simulink model "FOC"  (R2022a)
settings: Solver=VariableStepAuto  StartTime=0.0  StopTime=10.0  RelTol=1e-3
undefined symbols (not defined in the file): I_max, Ki_current, Kp_current, L_M_hat, magnitude, n_p, omega_1_N, psi_ref, R_R, R_R_hat, R_s, V_base, X_M_opt, X_sig_opt
libraries: eeTransforms x2, simulink x1, slpidlib x1
settings Model: Creator=Jakob  LastModifiedBy=Jakob

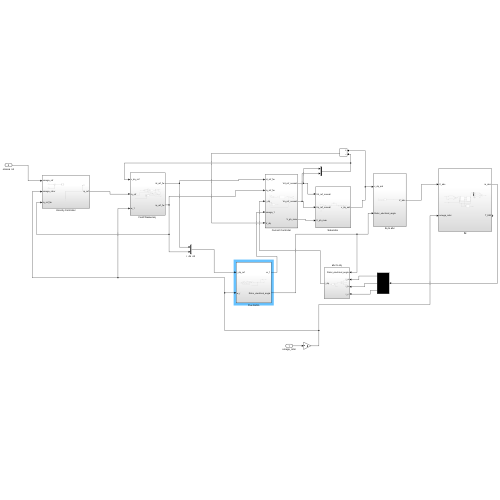
[thumbnail: Simulink's stored preview of the top-level diagram]
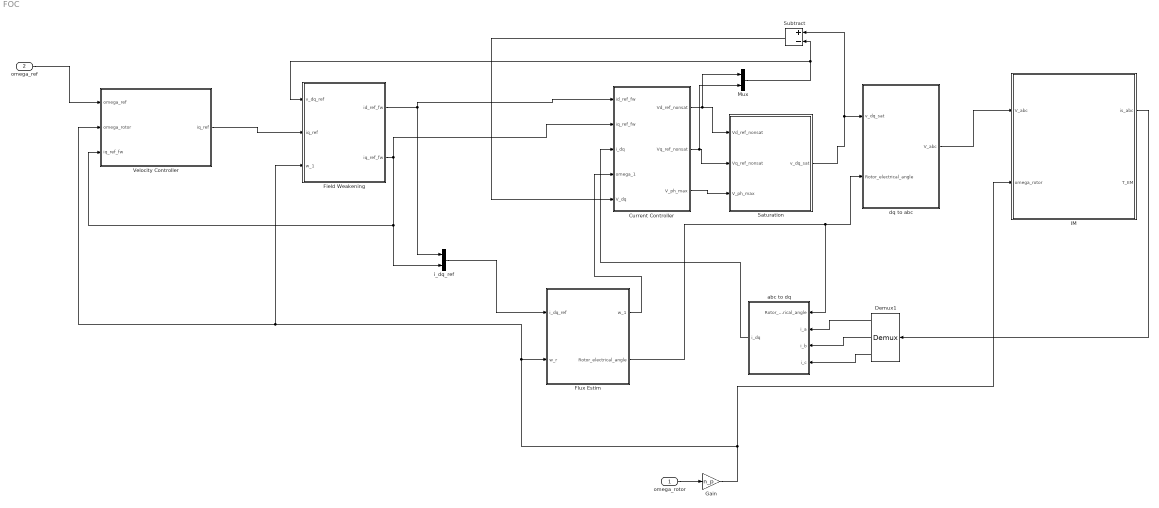
== system FOC ==
  omega_rotor : Inport
  omega_ref : Inport  Port=2
  Current Controller : Subsystem
  Demux1 : Demux  Outputs=3
  Field Weakening : Subsystem
  Flux Estim : Subsystem
  Gain : Gain  Gain=n_p
  IM : Subsystem
  Mux : Mux  Inputs=2
  Saturation : Subsystem
  Subtract : Sum  Inputs=+-
  Velocity Controller : Subsystem
  abc to dq : Subsystem
  dq to abc : Subsystem
  i_dq_ref : Mux  Inputs=2
  wires:
  dq to abc/1(V_abc) -> IM/1(V_abc)
  abc to dq/1(i_dq) -> Current Controller/3(i_dq)
  Current Controller/1(Vd_ref_nonsat) -> Mux/1, Saturation/1(Vd_ref_nonsat)
  Current Controller/2(Vq_ref_nonsat) -> Mux/2, Saturation/2(Vq_ref_nonsat)
  Current Controller/3(V_ph_max) -> Saturation/3(V_ph_max)
  Saturation/1(v_dq_sat) -> Subtract/1, dq to abc/1(v_dq_sat)
  Mux/1 -> Field Weakening/1(v_dq_ref), Subtract/2
  Subtract/1 -> Current Controller/5(V_dq)
  IM/1(is_abc) -> Demux1/1
  Demux1/1 -> abc to dq/2(i_a)
  Demux1/2 -> abc to dq/3(i_b)
  Demux1/3 -> abc to dq/4(i_c)
  omega_rotor/1 -> Gain/1
  omega_ref/1 -> Velocity Controller/1(omega_ref)
  Flux Estim/2(Rotor_electrical_angle) -> abc to dq/1(Rotor_electrical_angle), dq to abc/2(Rotor_electrical_angle)
  Flux Estim/1(w_1) -> Current Controller/4(omega_1)
  Gain/1 -> Flux Estim/2(w_r), Field Weakening/3(w_1), Velocity Controller/2(omega_rotor), IM/2(omega_rotor)
  Field Weakening/2(iq_ref_fw) -> Current Controller/2(iq_ref_fw), Velocity Controller/3(iq_ref_fw), i_dq_ref/2
  Velocity Controller/1(iq_ref) -> Field Weakening/2(iq_ref)
  Field Weakening/1(id_ref_fw) -> Current Controller/1(id_ref_fw), i_dq_ref/1
  i_dq_ref/1 -> Flux Estim/1(i_dq_ref)

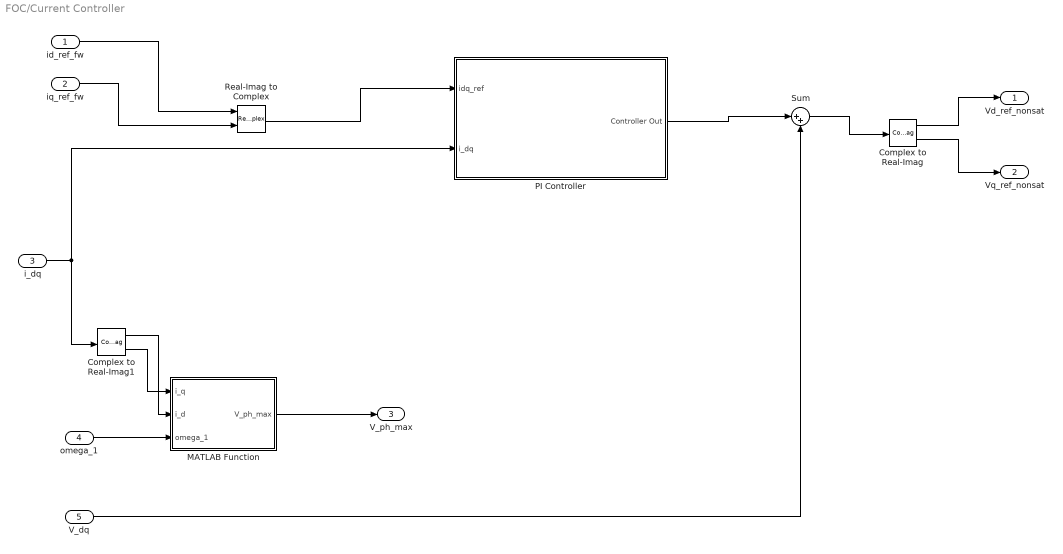
== system FOC/Current Controller ==
  id_ref_fw : Inport
  iq_ref_fw : Inport  Port=2
  i_dq : Inport  Port=3
  omega_1 : Inport  Port=4
  V_dq : Inport  Port=5
  Complex to Real-Imag : ComplexToRealImag
  Complex to Real-Imag1 : ComplexToRealImag
  MATLAB Function : MATLAB Function  TreatAsAtomicUnit=on
  PI Controller : Subsystem
  Real-Imag to Complex : RealImagToComplex
  Sum : Sum  Inputs=|++
  Vd_ref_nonsat : Outport
  Vq_ref_nonsat : Outport  Port=2
  V_ph_max : Outport  Port=3
  wires:
  i_dq/1 -> Complex to Real-Imag1/1, PI Controller/2(i_dq)
  Complex to Real-Imag1/1 -> MATLAB Function/2(i_d)
  Complex to Real-Imag1/2 -> MATLAB Function/1(i_q)
  omega_1/1 -> MATLAB Function/3(omega_1)
  id_ref_fw/1 -> Real-Imag to Complex/1
  iq_ref_fw/1 -> Real-Imag to Complex/2
  Real-Imag to Complex/1 -> PI Controller/1(idq_ref)
  PI Controller/1(Controller Out) -> Sum/1
  V_dq/1 -> Sum/2
  Sum/1 -> Complex to Real-Imag/1
  Complex to Real-Imag/1 -> Vd_ref_nonsat/1
  Complex to Real-Imag/2 -> Vq_ref_nonsat/1
  MATLAB Function/1(V_ph_max) -> V_ph_max/1

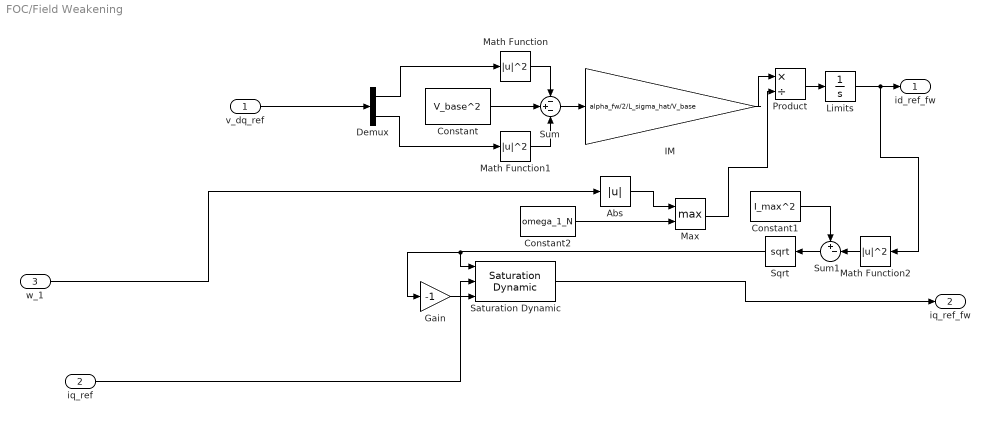
== system FOC/Field Weakening ==
  v_dq_ref : Inport
  iq_ref : Inport  Port=2
  w_1 : Inport  Port=3
  Abs : Abs  SaturateOnIntegerOverflow=off
  Constant : Constant  Value=V_base^2
  Constant1 : Constant  Value=I_max^2
  Constant2 : Constant  Value=omega_1_N
  Demux : Demux  Outputs=2
  Gain : Gain  Gain=-1
  IM : Gain  Gain=alpha_fw/2/L_sigma_hat/V_base
  Limits : Integrator  LimitOutput=on  UpperSaturationLimit=psi_ref/L_M_hat  LowerSaturationLimit=0.1*psi_ref/L_M_hat
  Math Function : Math  Operator=magnitude^2
  Math Function1 : Math  Operator=magnitude^2
  Math Function2 : Math  Operator=magnitude^2
  Max : MinMax  Function=max  Inputs=2
  Product : Product  Inputs=*/
  Saturation Dynamic : simulink/Discontinuities/Saturation Dynamic  OutMin=[]  OutMax=[]  OutDataTypeStr=Inherit: Same as second input  OutDataType=fixdt(1, 16)  OutScaling=2^-10  DoSatur=off
  Sqrt : Sqrt
  Sum : Sum  Inputs=-+-
  Sum1 : Sum  Inputs=+-|
  id_ref_fw : Outport
  iq_ref_fw : Outport  Port=2
  wires:
  Abs/1 -> Max/1
  Sum1/1 -> Sqrt/1
  Max/1 -> Product/2
  Math Function2/1 -> Sum1/2
  w_1/1 -> Abs/1
  v_dq_ref/1 -> Demux/1
  Math Function1/1 -> Sum/3
  Product/1 -> Limits/1
  Sqrt/1 -> Gain/1, Saturation Dynamic/1
  Gain/1 -> Saturation Dynamic/3
  Constant1/1 -> Sum1/1
  Constant2/1 -> Max/2
  Saturation Dynamic/1 -> iq_ref_fw/1
  Demux/2 -> Math Function1/1
  Limits/1 -> id_ref_fw/1, Math Function2/1
  Math Function/1 -> Sum/1
  IM/1 -> Product/1
  Sum/1 -> IM/1
  iq_ref/1 -> Saturation Dynamic/2
  Constant/1 -> Sum/2
  Demux/1 -> Math Function/1

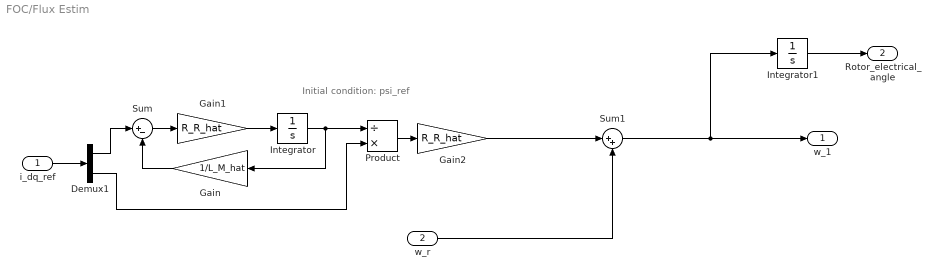
== system FOC/Flux Estim ==
  note: Initial condition: psi_ref
  i_dq_ref : Inport
  w_r : Inport  Port=2
  Demux1 : Demux  Outputs=2
  Gain : Gain  Gain=1/L_M_hat
  Gain1 : Gain  Gain=R_R_hat
  Gain2 : Gain  Gain=R_R_hat
  Integrator : Integrator  InitialCondition=psi_ref
  Integrator1 : Integrator
  Product : Product  Inputs=/*
  Sum : Sum  Inputs=|+-
  Sum1 : Sum  Inputs=|++
  w_1 : Outport
  Rotor_electrical_angle : Outport  Port=2
  wires:
  Gain1/1 -> Integrator/1
  Sum1/1 -> Integrator1/1, w_1/1
  Product/1 -> Gain2/1
  i_dq_ref/1 -> Demux1/1
  Demux1/1 -> Sum/1
  Demux1/2 -> Product/2
  Integrator/1 -> Gain/1, Product/1
  Gain/1 -> Sum/2
  Sum/1 -> Gain1/1
  Gain2/1 -> Sum1/1
  w_r/1 -> Sum1/2
  Integrator1/1 -> Rotor_electrical_angle/1

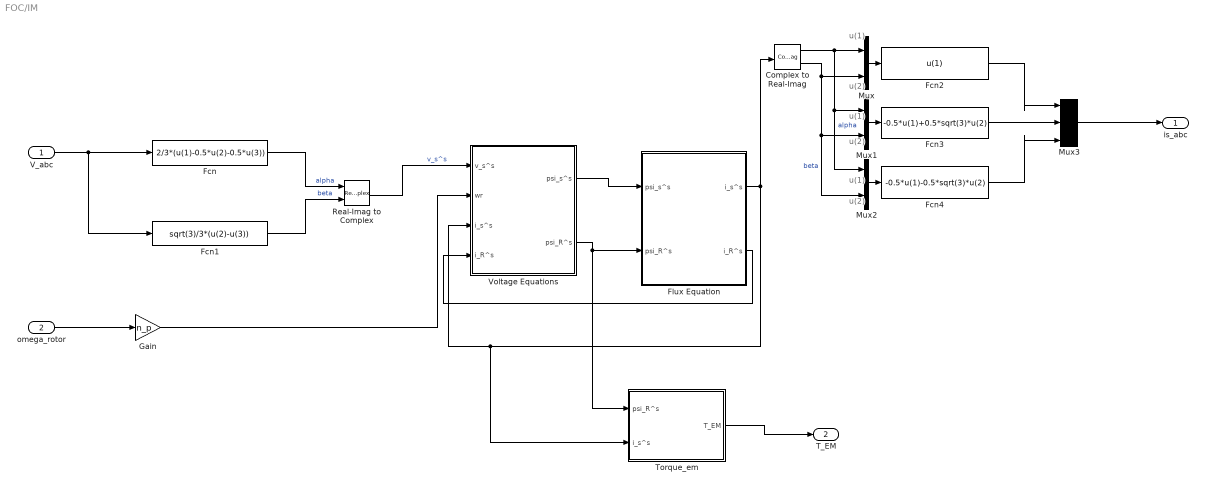
== system FOC/IM ==
  note: u(1)
  note: u(2)
  note: u(2)
  note: u(2)
  note: u(1)
  note: u(1)
  V_abc : Inport
  omega_rotor : Inport  Port=2
  Complex to Real-Imag : ComplexToRealImag
  Fcn : Fcn  Expr=2/3*(u(1)-0.5*u(2)-0.5*u(3))
  Fcn1 : Fcn  Expr=sqrt(3)/3*(u(2)-u(3))
  Fcn2 : Fcn  Expr=u(1)
  Fcn3 : Fcn  Expr=-0.5*u(1)+0.5*sqrt(3)*u(2)
  Fcn4 : Fcn  Expr=-0.5*u(1)-0.5*sqrt(3)*u(2)
  Flux Equation : Subsystem
  Gain : Gain  Gain=n_p
  Mux : Mux  Inputs=2
  Mux1 : Mux  Inputs=2
  Mux2 : Mux  Inputs=2
  Mux3 : Mux  Inputs=3
  Real-Imag to Complex : RealImagToComplex
  Torque_em : Subsystem
  Voltage Equations : Subsystem
  is_abc : Outport
  T_EM : Outport  Port=2
  wires:
  V_abc/1 -> Fcn1/1, Fcn/1
  Fcn/1 -> Real-Imag to Complex/1  "alpha"
  Fcn1/1 -> Real-Imag to Complex/2  "beta"
  Real-Imag to Complex/1 -> Voltage Equations/1(v_s^s)  "v_s^s"
  omega_rotor/1 -> Gain/1
  Gain/1 -> Voltage Equations/2(wr)
  Voltage Equations/1(psi_s^s) -> Flux Equation/1(psi_s^s)
  Voltage Equations/2(psi_R^s) -> Torque_em/1(psi_R^s), Flux Equation/2(psi_R^s)
  Complex to Real-Imag/1 -> Mux2/1, Mux1/1, Mux/1  "alpha"
  Mux/1 -> Fcn2/1
  Complex to Real-Imag/2 -> Mux2/2, Mux1/2, Mux/2  "beta"
  Mux2/1 -> Fcn4/1
  Flux Equation/1(i_s^s) -> Complex to Real-Imag/1, Torque_em/2(i_s^s), Voltage Equations/3(i_s^s)
  Mux1/1 -> Fcn3/1
  Fcn4/1 -> Mux3/3
  Fcn3/1 -> Mux3/2
  Fcn2/1 -> Mux3/1
  Mux3/1 -> is_abc/1
  Flux Equation/2(i_R^s) -> Voltage Equations/4(i_R^s)
  Torque_em/1(T_EM) -> T_EM/1

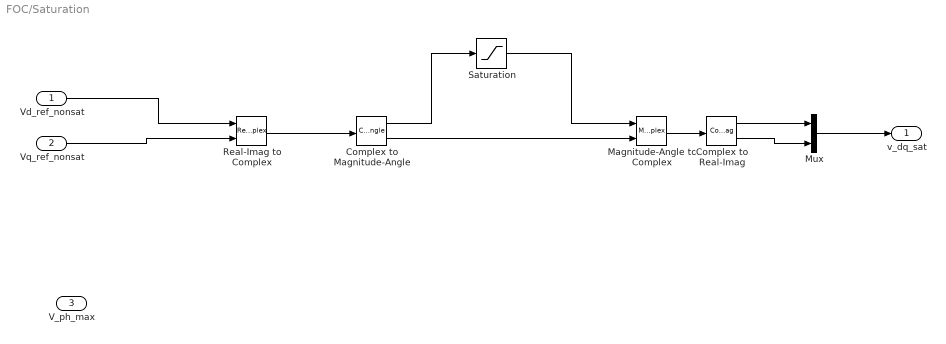
== system FOC/Saturation ==
  Vd_ref_nonsat : Inport
  Vq_ref_nonsat : Inport  Port=2
  V_ph_max : Inport  Port=3
  Complex to Magnitude-Angle : ComplexToMagnitudeAngle
  Complex to Real-Imag : ComplexToRealImag
  Magnitude-Angle to Complex : MagnitudeAngleToComplex
  Mux : Mux  Inputs=2
  Real-Imag to Complex : RealImagToComplex
  Saturation : Saturate  UpperLimit=400/sqrt(3) * sqrt(2)  LowerLimit=0
  v_dq_sat : Outport
  wires:
  Vd_ref_nonsat/1 -> Real-Imag to Complex/1
  Vq_ref_nonsat/1 -> Real-Imag to Complex/2
  Real-Imag to Complex/1 -> Complex to Magnitude-Angle/1
  Complex to Magnitude-Angle/1 -> Saturation/1
  Saturation/1 -> Magnitude-Angle to Complex/1
  Complex to Magnitude-Angle/2 -> Magnitude-Angle to Complex/2
  Magnitude-Angle to Complex/1 -> Complex to Real-Imag/1
  Complex to Real-Imag/1 -> Mux/1
  Complex to Real-Imag/2 -> Mux/2
  Mux/1 -> v_dq_sat/1

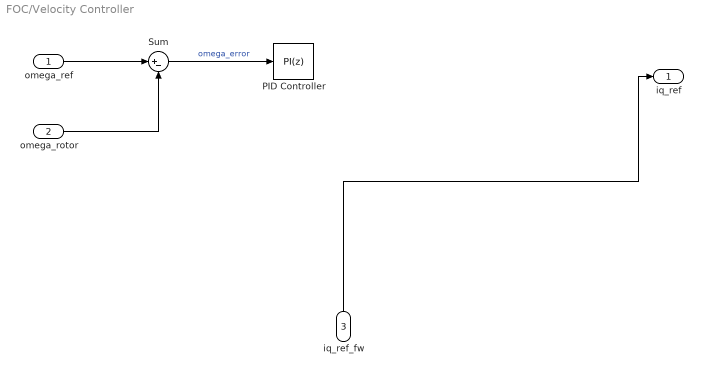
== system FOC/Velocity Controller ==
  omega_ref : Inport
  omega_rotor : Inport  Port=2
  iq_ref_fw : Inport  Port=3
  PID Controller : slpidlib/PID Controller  Controller=PI  Form=Parallel  TimeDomain=Discrete-time  UseExternalTs=off  SampleTime=-1  IntegratorMethod=Forward Euler  FilterMethod=Forward Euler  ControllerParametersSource=internal  P=1  I=1  UseKiTs=off  D=0  N=100  UseFilter=on  TunerSelectOption=Transfer Function Based (PID Tuner App)  InitialConditionSource=internal  InitialConditionForIntegrator=0  InitialConditionForFilter=0  DifferentiatorICPrevScaledInput=0  ExternalReset=none  TrackingMode=off  Kt=1  LimitOutput=off  SatLimitsSource=internal  UpperSaturationLimit=inf  LowerSaturationLimit=-inf  LinearizeAsGain=on  AntiWindupMode=none  Kb=1  POutMin=[]  POutMax=[]  IOutMin=[]  IOutMax=[]  DOutMin=[]  DOutMax=[]  NOutMin=[]  NOutMax=[]  SumOutMin=[]  SumOutMax=[]  SaturationOutMin=[]  SaturationOutMax=[]  PParamMin=[]  PParamMax=[]  IParamMin=[]  IParamMax=[]  DParamMin=[]  DParamMax=[]  NParamMin=[]  NParamMax=[]  KbParamMin=[]  KbParamMax=[]  KtParamMin=[]  KtParamMax=[]  KbOutMin=[]  KbOutMax=[]  KtOutMin=[]  KtOutMax=[]  IntegratorOutMin=[]  IntegratorOutMax=[]  FilterOutMin=[]  FilterOutMax=[]  SumI1OutMin=[]  SumI1OutMax=[]  SumI2OutMin=[]  SumI2OutMax=[]  SumI3OutMin=[]  SumI3OutMax=[]  SumI4OutMin=[]  SumI4OutMax=[]  SumDOutMin=[]  SumDOutMax=[]  DifferentiatorOutMin=[]  DifferentiatorOutMax=[]  FilterDiffOutCoefMin=[]  FilterDiffOutCoefMax=[]  ReciprocalOutMin=[]  ReciprocalOutMax=[]  SumDenOutMin=[]  SumDenOutMax=[]  SumNumOutMin=[]  SumNumOutMax=[]  DivideOutMin=[]  DivideOutMax=[]  UdiffTsProdOutMin=[]  UdiffTsProdOutMax=[]  NTsProdOutMin=[]  NTsProdOutMax=[]  UintegralTsProdOutMin=[]  UintegralTsProdOutMax=[]  UngainTsProdOutMin=[]  UngainTsProdOutMax=[]  IntegratorContinuousStateAttributes=''  IntegratorStateMustResolveToSignalObject=off  IntegratorRTWStateStorageClass=Auto  FilterContinuousStateAttributes=''  FilterStateMustResolveToSignalObject=off  FilterRTWStateStorageClass=Auto  ParallelPVariant=InternalParameters  IdealPVariant=Disabled  IVariant=InternalParameters  DVariant=Disabled  IntegratorVariant=Discrete  SatVariant=Disabled  AWVariant=Passthrough  PCopyVariant=Disabled  TRVariant=Disabled  FdbkBlocksVariant=Forward  IdealPFdbkVariant=Disabled  SatFdbkVariant=Disabled  DerivativeFilterVariant=Disabled  NVariant=Disabled  NCopyVariant=Disabled_SignalSpec  FilterICVariant=Disabled  IntegratorICVariant=InternalICs  ExternalResetVariant=Disabled  TRSumVariant=Passthrough  SumFdbkVariant=Disabled  SumVariant=Sum_PI  TsampFilterVariant=InternalTs  TsampNgainVariant=Passthrough  TsampIntegralVariant=Passthrough  ExternalSaturationOutDataTypeStr=Inherit: Same as second input  aMode=0
  Sum : Sum  Inputs=|+-
  iq_ref : Outport
  wires:
  omega_ref/1 -> Sum/1
  omega_rotor/1 -> Sum/2
  Sum/1 -> PID Controller/1  "omega_error"
  iq_ref_fw/1 -> iq_ref/1

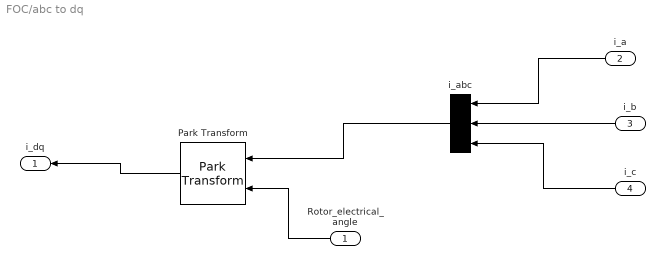
== system FOC/abc to dq ==
  Rotor_electrical_angle : Inport
  i_a : Inport  Port=2
  i_b : Inport  Port=3
  i_c : Inport  Port=4
  Park Transform : eeTransforms/Park Transform  AxisAlignment=Q-axis  PowerInvariant=off
  i_abc : Mux  Inputs=3
  i_dq : Outport
  wires:
  i_abc/1 -> Park Transform/1
  i_c/1 -> i_abc/3
  i_b/1 -> i_abc/2
  i_a/1 -> i_abc/1
  Rotor_electrical_angle/1 -> Park Transform/2
  Park Transform/1 -> i_dq/1

== system FOC/dq to abc ==
  v_dq_sat : Inport
  Rotor_electrical_angle : Inport  Port=2
  Inverse Park Transform : eeTransforms/Inverse Park Transform  AxisAlignment=Q-axis  PowerInvariant=off
  V_abc : Outport
  wires:
  v_dq_sat/1 -> Inverse Park Transform/1
  Inverse Park Transform/1 -> V_abc/1
  Rotor_electrical_angle/1 -> Inverse Park Transform/2

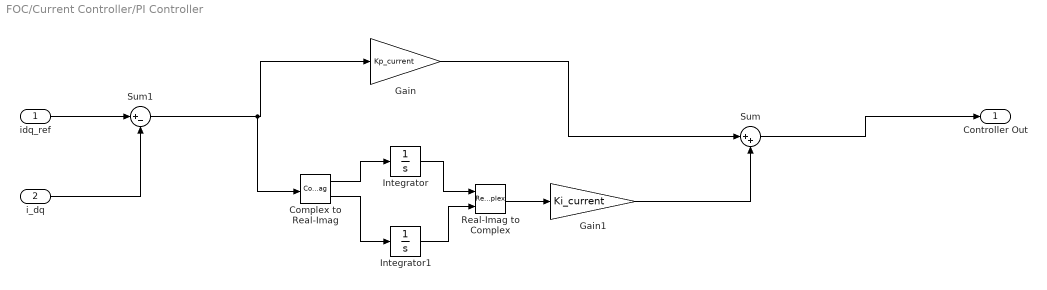
== system FOC/Current Controller/PI Controller ==
  idq_ref : Inport
  i_dq : Inport  Port=2
  Complex to Real-Imag : ComplexToRealImag
  Gain : Gain  Gain=Kp_current
  Gain1 : Gain  Gain=Ki_current
  Integrator : Integrator
  Integrator1 : Integrator
  Real-Imag to Complex : RealImagToComplex
  Sum : Sum  Inputs=|++
  Sum1 : Sum  Inputs=|+-
  Controller Out : Outport
  wires:
  Complex to Real-Imag/1 -> Integrator/1
  Complex to Real-Imag/2 -> Integrator1/1
  Integrator/1 -> Real-Imag to Complex/1
  Integrator1/1 -> Real-Imag to Complex/2
  Real-Imag to Complex/1 -> Gain1/1
  Gain/1 -> Sum/1
  Gain1/1 -> Sum/2
  Sum/1 -> Controller Out/1
  idq_ref/1 -> Sum1/1
  i_dq/1 -> Sum1/2
  Sum1/1 -> Complex to Real-Imag/1, Gain/1

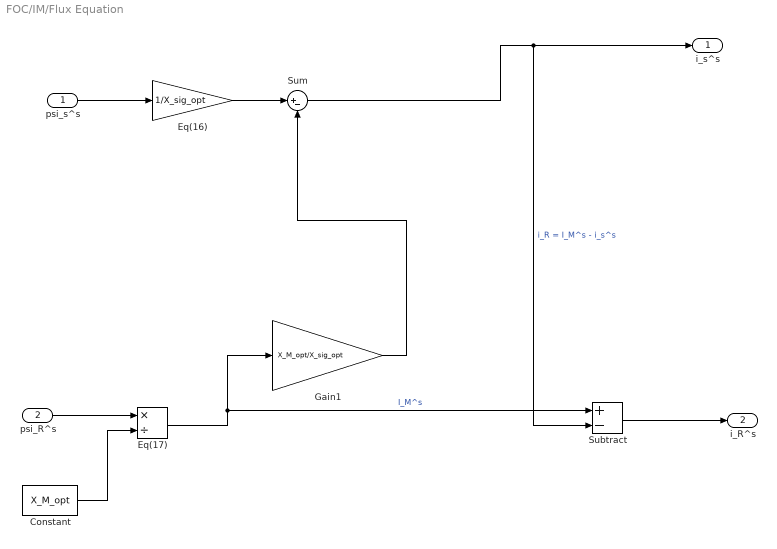
== system FOC/IM/Flux Equation ==
  psi_s^s : Inport
  psi_R^s : Inport  Port=2
  Constant : Constant  Value=X_M_opt
  Eq(16) : Gain  Gain=1/X_sig_opt
  Eq(17) : Product  Inputs=*/
  Gain1 : Gain  Gain=X_M_opt/X_sig_opt
  Subtract : Sum  Inputs=+-
  Sum : Sum  Inputs=|+-
  i_s^s : Outport
  i_R^s : Outport  Port=2
  wires:
  psi_s^s/1 -> Eq(16)/1
  Eq(16)/1 -> Sum/1
  Sum/1 -> Subtract/2, i_s^s/1  "i_R = I_M^s - i_s^s"
  psi_R^s/1 -> Eq(17)/1
  Constant/1 -> Eq(17)/2
  Eq(17)/1 -> Subtract/1, Gain1/1  "I_M^s"
  Gain1/1 -> Sum/2
  Subtract/1 -> i_R^s/1

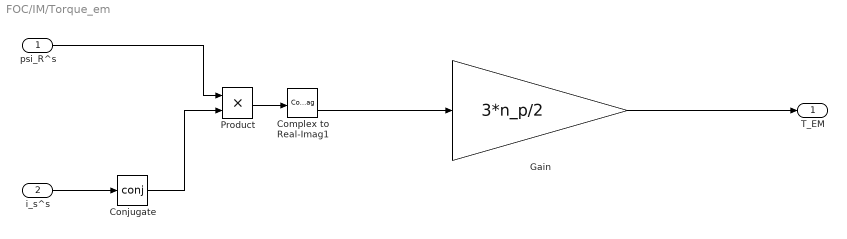
== system FOC/IM/Torque_em ==
  psi_R^s : Inport
  i_s^s : Inport  Port=2
  Complex to Real-Imag1 : ComplexToRealImag
  Conjugate : Math  Operator=conj  SignedPower=on  RndMeth=Zero
  Gain : Gain  Gain=3*n_p/2
  Product : Product
  T_EM : Outport
  wires:
  i_s^s/1 -> Conjugate/1
  psi_R^s/1 -> Product/1
  Conjugate/1 -> Product/2
  Product/1 -> Complex to Real-Imag1/1
  Complex to Real-Imag1/2 -> Gain/1
  Gain/1 -> T_EM/1

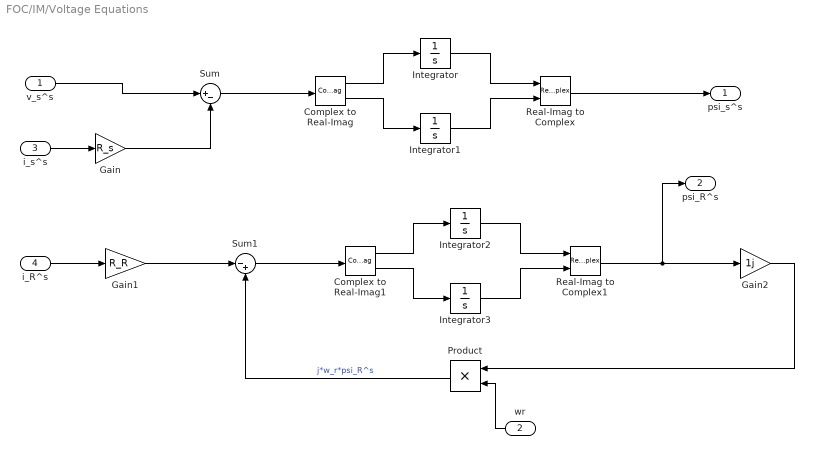
== system FOC/IM/Voltage Equations ==
  v_s^s : Inport
  wr : Inport  Port=2
  i_s^s : Inport  Port=3
  i_R^s : Inport  Port=4
  Complex to Real-Imag : ComplexToRealImag
  Complex to Real-Imag1 : ComplexToRealImag
  Gain : Gain  Gain=R_s
  Gain1 : Gain  Gain=R_R
  Gain2 : Gain  Gain=1j
  Integrator{,1..3} (4 alike) : Integrator
  Product : Product
  Real-Imag to Complex : RealImagToComplex
  Real-Imag to Complex1 : RealImagToComplex
  Sum : Sum  Inputs=|+-
  Sum1 : Sum  Inputs=|-+
  psi_s^s : Outport
  psi_R^s : Outport  Port=2
  wires:
  v_s^s/1 -> Sum/1
  i_s^s/1 -> Gain/1
  Gain/1 -> Sum/2
  Sum/1 -> Complex to Real-Imag/1
  Complex to Real-Imag/1 -> Integrator/1
  Complex to Real-Imag/2 -> Integrator1/1
  Integrator/1 -> Real-Imag to Complex/1
  Integrator1/1 -> Real-Imag to Complex/2
  Real-Imag to Complex/1 -> psi_s^s/1
  i_R^s/1 -> Gain1/1
  Gain1/1 -> Sum1/1
  Complex to Real-Imag1/2 -> Integrator3/1
  Integrator2/1 -> Real-Imag to Complex1/1
  Integrator3/1 -> Real-Imag to Complex1/2
  Real-Imag to Complex1/1 -> psi_R^s/1, Gain2/1
  Complex to Real-Imag1/1 -> Integrator2/1
  Sum1/1 -> Complex to Real-Imag1/1
  wr/1 -> Product/2
  Gain2/1 -> Product/1
  Product/1 -> Sum1/2  "j*w_r*psi_R^s"

== matlab function FOC/Current Controller/MATLAB Function ==
  data: i_q input; V_ph_max output; i_d input; omega_1 input
function V_ph_max = fcn(i_q, i_d, omega_1)

V_ph_max = abs(omega_1)*L_sigma*sqrt((i_q)^2 + ((L_sigma + L_M)/L_sigma)^2 * i_d^2);
